simulink model "mpc1_sim"  (R2020a)
settings: Solver=VariableStepAuto  StartTime=0.0  StopTime=1000  RelTol=1e-3
values from neighbouring files (symbols this model uses):
  Ts = 0.1    [data_mpc.mat]    (also in so_priklad.m)
libraries: mpclib x2, cstblocks x2
settings Model: Creator=mgoubej  LastModifiedBy=mgoubej

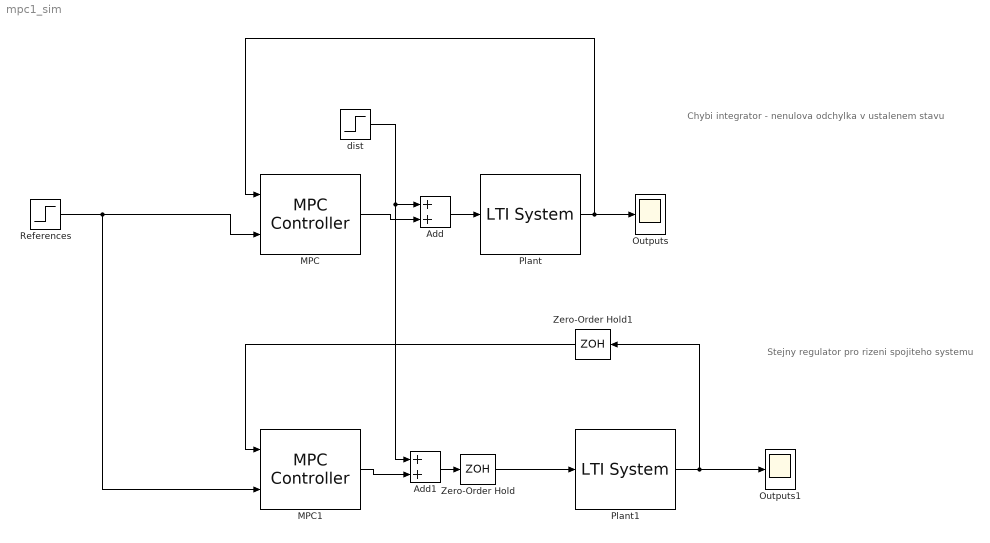
== system mpc1_sim ==
  note: Stejny regulator pro rizeni spojiteho systemu
  note: Chybi integrator - nenulova odchylka v ustalenem stavu
  Add : Sum
  Add1 : Sum
  MPC : mpclib/MPC Controller  SCDEnableBlockLinearizationSpecification=on  mpcobj=mpc1  is_multiple=0  enable_value=0  return_u0=off  updateMPCinCallerWorkspace=on  md_inport=off  mv_inport=off  uref_inport=off  return_cost=off  return_mvseq=off  return_qpstatus=off  return_xseq=off  return_state=off  return_ovseq=off  state_inport=off  umin_inport=off  umax_inport=off  ymin_inport=off  ymax_inport=off  cc_inport=off  ywt_inport=off  uwt_inport=off  duwt_inport=off  rhoeps_inport=off  pm_inport=off  MaximumP=10  HorizonChoice=FixedHorizon  n_ts=0.1  n_p=10  n_mv=1  n_md=0  n_ud=0  n_mo=1  n_uo=0  BlockDataType=double  SampleTimeInherited=off  switch_inport=off
  MPC1 : mpclib/MPC Controller  SCDEnableBlockLinearizationSpecification=on  mpcobj=mpc1  is_multiple=0  enable_value=0  return_u0=off  updateMPCinCallerWorkspace=on  md_inport=off  mv_inport=off  uref_inport=off  return_cost=off  return_mvseq=off  return_qpstatus=off  return_xseq=off  return_state=off  return_ovseq=off  state_inport=off  umin_inport=off  umax_inport=off  ymin_inport=off  ymax_inport=off  cc_inport=off  ywt_inport=off  uwt_inport=off  duwt_inport=off  rhoeps_inport=off  pm_inport=off  MaximumP=10  HorizonChoice=FixedHorizon  n_ts=0.1  n_p=10  n_mv=1  n_md=0  n_ud=0  n_mo=1  n_uo=0  BlockDataType=double  SampleTimeInherited=off  switch_inport=off
  Outputs : Scope
  Outputs1 : Scope
  Plant : cstblocks/LTI System  sys=Pss  IC=[]
  Plant1 : cstblocks/LTI System  sys=P  IC=[]
  References : Step
  Zero-Order Hold : ZeroOrderHold  SampleTime=Ts
  Zero-Order Hold1 : ZeroOrderHold  SampleTime=Ts
  dist : Step  Time=5  After=0.1
  wires:
  References/1 -> MPC1/2, MPC/2
  Plant/1 -> MPC/1, Outputs/1
  Add/1 -> Plant/1
  MPC/1 -> Add/2
  dist/1 -> Add1/1, Add/1
  MPC1/1 -> Add1/2
  Add1/1 -> Zero-Order Hold/1
  Zero-Order Hold/1 -> Plant1/1
  Plant1/1 -> Zero-Order Hold1/1, Outputs1/1
  Zero-Order Hold1/1 -> MPC1/1
